simulink model "a3"  (Simulink 8.7)
settings: Solver=VariableStepAuto  StartTime=0.0  StopTime=1000  RelTol=1e-3
libraries: vrlib x2
settings Model: Creator=Birger  LastModifiedBy=Birger
settings DataIOCC: LimitDataPoints=off  SaveFormat=Dataset
settings DebuggingCC: UnderspecifiedInitializationDetection=Simplified  MergeDetectMultiDrivingBlocksExec=error
settings HardwareCC: ProdBitPerPointer=64  ProdLargestAtomicFloat=Float  ProdIntDivRoundTo=Zero  ProdEndianess=LittleEndian  ProdWordSize=64  ProdHWDeviceType=Intel->x86-64 (Windows64)
settings ModelReferenceCC: PropagateSignalLabelsOutOfModel=on
settings ConfigComp: CovModelRefEnable=off

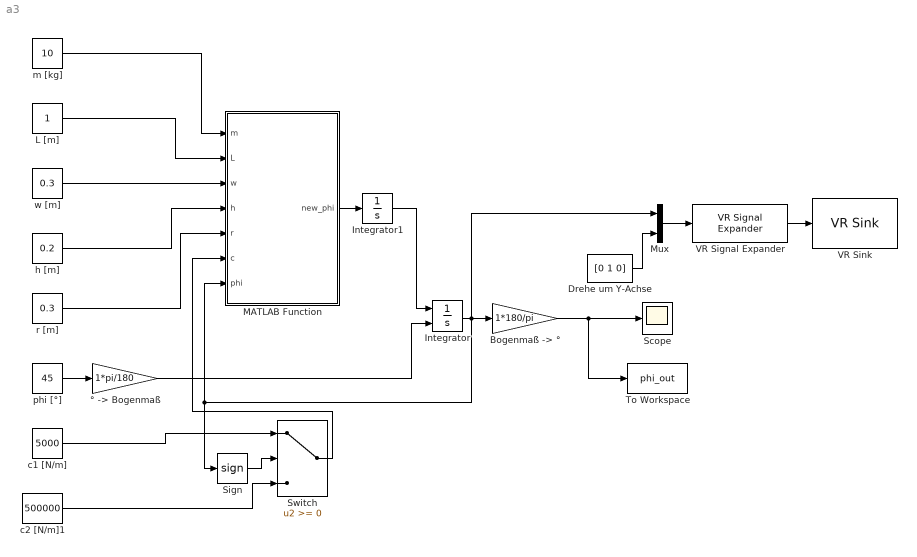
== system a3 ==
  "Bogenmaß -> °" : Gain  Gain=1*180/pi
  Drehe um Y-Achse : Constant  Value=[0 1 0]
  Integrator : Integrator  InitialConditionSource=external
  Integrator1 : Integrator
  L [m] : Constant
  MATLAB Function : MATLAB Function  TreatAsAtomicUnit=on
  Mux : Mux  Inputs=2
  Scope : Scope
  Sign : Signum
  Switch : Switch
  To Workspace : ToWorkspace  VariableName=phi_out  SaveFormat=Timeseries  SampleTime=-1
  VR Signal Expander : vrlib/VR Signal Expander  outwidth=4  outidx=[4 1 2 3]
  VR Sink : vrlib/VR Sink  InstantiateOnLoad=on  SampleTime=0.005  ViewEnable=on  RemoteChange=off  RemoteView=on  FieldsWritten=Seiltrommel.rotation.4.1.1.double  WorldFileName=CrazyPendlm.wrl  AutoView=off  VideoDimensions=[]  AllowVariableSize=off
  c1 [N/m] : Constant  Value=5000
  c2 [N/m]1 : Constant  Value=500000
  h [m] : Constant  Value=0.2
  m [kg] : Constant  Value=10
  phi [°] : Constant  Value=45
  r [m] : Constant  Value=0.3
  w [m] : Constant  Value=0.3
  "° -> Bogenmaß" : Gain  Gain=1*pi/180
  wires:
  c1 [N/m]/1 -> Switch/1
  c2 [N/m]1/1 -> Switch/3
  w [m]/1 -> MATLAB Function/3(w)
  L [m]/1 -> MATLAB Function/2(L)
  m [kg]/1 -> MATLAB Function/1(m)
  h [m]/1 -> MATLAB Function/4(h)
  r [m]/1 -> MATLAB Function/5(r)
  Switch/1 -> MATLAB Function/6(c)
  Sign/1 -> Switch/2
  MATLAB Function/1(new_phi) -> Integrator1/1
  phi [°]/1 -> "° -> Bogenmaß"/1
  Integrator1/1 -> Integrator/1
  Drehe um Y-Achse/1 -> Mux/2
  Mux/1 -> VR Signal Expander/1
  VR Signal Expander/1 -> VR Sink/1
  Integrator/1 -> "Bogenmaß -> °"/1, Sign/1, MATLAB Function/7(phi), Mux/1
  "° -> Bogenmaß"/1 -> Integrator/2
  "Bogenmaß -> °"/1 -> To Workspace/1, Scope/1

== matlab function MATLAB Function ==
  data: m input double; new_phi output double; L input double; w input double; h input double; r input double; c input double; phi input double
function new_phi = fcn(m,L,w,h,r,c,phi)
%#codegen

g=9.80665; %m/s^2

Mp = m*g*sin(phi)*(L+h/2);
Ms = -phi * c * r^2;
Mg = Mp + Ms;

Jp = 1/12 * m *(h^2 + w^2);
Jg = Jp + m*(L + h/2)^2;

new_phi = Mg/Jg;
